simulink model "lab1_simu"  (R2024b)
settings: Solver=VariableStepAuto  StartTime=0.0  StopTime=30  RelTol=1e-3
values from neighbouring files (symbols this model uses):
  A = [0 1 0 0 ... (first row only)    [code_cte_small.m]    (also in lab1.m)
  Afcc = inv(T) * A * T    [code_cte_small.m]    (also in lab1.m)
  Afco = inv(Q)*A*Q    [code_cte_small.m]    (also in lab1.m)
  B = [0 ... (first row only)    [code_cte_small.m]    (also in lab1.m)
  Bfcc = inv(T) * B    [code_cte_small.m]    (also in lab1.m)
  Bfco = inv(Q) * B    [code_cte_small.m]    (also in lab1.m)
  C = [1 0 0 0]    [code_cte_small.m]    (also in lab1.m)
  Cfcc = C * T    [code_cte_small.m]    (also in lab1.m)
  Cfco = C * Q    [code_cte_small.m]    (also in lab1.m)
  E = [0 ... (first row only)    [code_cte_small.m]    (also in lab1.m)
  Efcc = inv(T)*E    [code_cte_small.m]    (also in lab1.m)
  Efco = inv(Q) * E    [code_cte_small.m]    (also in lab1.m)
  KA = [-19.21, 9.68, 4.10, -15.739]    [code_cte_small.m]    (also in lab1.m = [-46190/327, 28467610/962361, -3048419/32700, 2598423281/481)
  KAfcc = [-29798.327,25528.529, 7395.9961,14.998605]    [code_cte_small.m]    (also in lab1.m = [-22691668,516984.21, -10797.714,-24.42])
  kiA = -24.76    [code_cte_small.m]    (also in lab1.m = 67.9102956167)
  kiAfcc = [-151.09413]    [code_cte_small.m]    (also in lab1.m = [67.910289])
settings Model: Creator=Acer  LastModifiedBy=Usuario

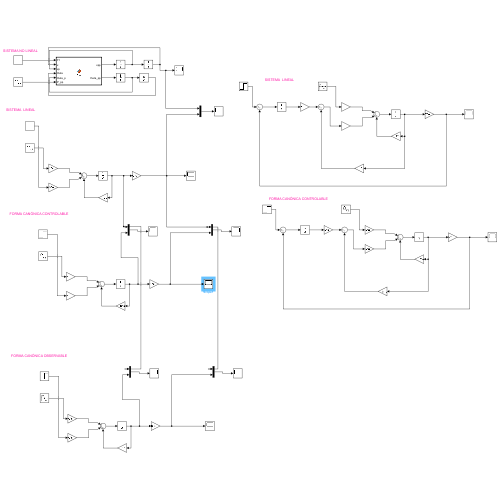
[thumbnail: Simulink's stored preview of the top-level diagram]
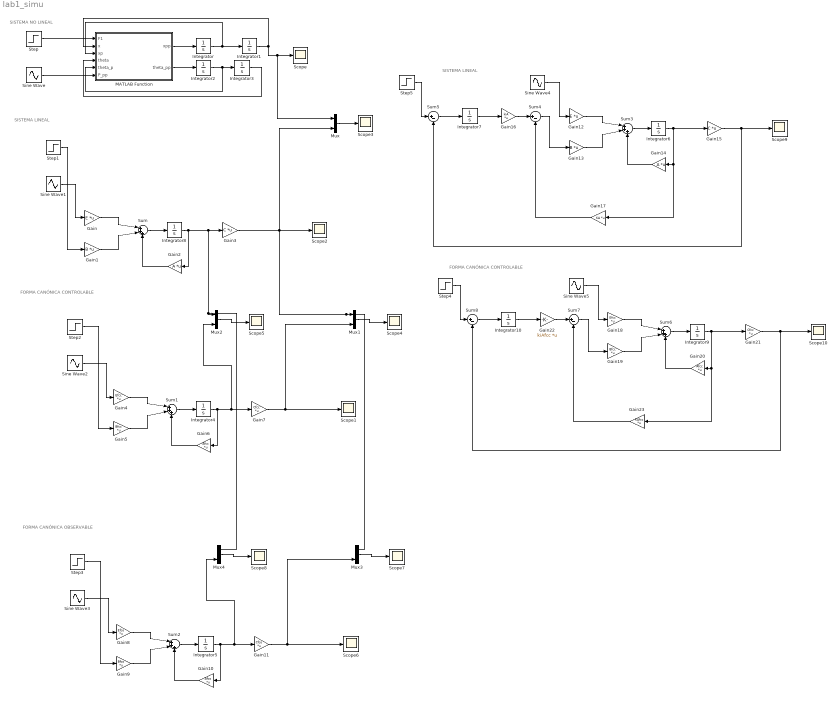
== system lab1_simu ==
  note: SISTEMA LINEAL
  note: SISTEMA NO LINEAL
  note: FORMA CANÓNICA CONTROLABLE
  note: FORMA CANÓNICA OBSERVABLE
  note: SISTEMA LINEAL
  note: FORMA CANÓNICA CONTROLABLE
  Gain : Gain  Gain=E  Multiplication=Matrix(K*u)
  Gain1 : Gain  Gain=B  Multiplication=Matrix(K*u)
  Gain10 : Gain  Gain=Afco  Multiplication=Matrix(K*u)
  Gain11 : Gain  Gain=Cfco  Multiplication=Matrix(K*u)
  Gain12 : Gain  Gain=E  Multiplication=Matrix(K*u)
  Gain13 : Gain  Gain=B  Multiplication=Matrix(K*u)
  Gain14 : Gain  Gain=A  Multiplication=Matrix(K*u)
  Gain15 : Gain  Gain=C  Multiplication=Matrix(K*u)
  Gain16 : Gain  Gain=kiA  Multiplication=Matrix(K*u)
  Gain17 : Gain  Gain=KA  Multiplication=Matrix(K*u)
  Gain18 : Gain  Gain=Efcc  Multiplication=Matrix(K*u)
  Gain19 : Gain  Gain=Bfcc  Multiplication=Matrix(K*u)
  Gain2 : Gain  Gain=A  Multiplication=Matrix(K*u)
  Gain20 : Gain  Gain=Afcc  Multiplication=Matrix(K*u)
  Gain21 : Gain  Gain=Cfcc  Multiplication=Matrix(K*u)
  Gain22 : Gain  Gain=kiAfcc  Multiplication=Matrix(K*u)
  Gain23 : Gain  Gain=KAfcc  Multiplication=Matrix(K*u)
  Gain3 : Gain  Gain=C  Multiplication=Matrix(K*u)
  Gain4 : Gain  Gain=Efcc  Multiplication=Matrix(K*u)
  Gain5 : Gain  Gain=Bfcc  Multiplication=Matrix(K*u)
  Gain6 : Gain  Gain=Afcc  Multiplication=Matrix(K*u)
  Gain7 : Gain  Gain=Cfcc  Multiplication=Matrix(K*u)
  Gain8 : Gain  Gain=Efco  Multiplication=Matrix(K*u)
  Gain9 : Gain  Gain=Bfco  Multiplication=Matrix(K*u)
  Integrator{,1..10} (11 alike) : Integrator
  MATLAB Function : MATLAB Function  TreatAsAtomicUnit=on
  Mux{,1..4} (5 alike) : Mux  Inputs=2
  Scope{,1..10} (11 alike) : Scope
  Sine Wave{,1..5} (6 alike) : Sin  Frequency=5  SampleTime=0
  Step{,1..5} (6 alike) : Step  Time=0  SampleTime=0
  Sum{,1..3,6} (5 alike) : Sum  Inputs=|+++
  Sum{4..5,7..8} (4 alike) : Sum  Inputs=|+-
  wires:
  MATLAB Function/1(xpp) -> Integrator/1
  Integrator/1 -> Integrator1/1, MATLAB Function/3(xp)
  Integrator1/1 -> MATLAB Function/2(x), Mux/1, Scope/1
  MATLAB Function/2(theta_pp) -> Integrator2/1
  Integrator2/1 -> Integrator3/1, MATLAB Function/5(theta_p)
  Integrator3/1 -> MATLAB Function/4(theta)
  Sine Wave/1 -> MATLAB Function/6(P_pp)
  Step/1 -> MATLAB Function/1(F1)
  Step1/1 -> Gain1/1
  Sine Wave1/1 -> Gain/1
  Gain/1 -> Sum/1
  Gain1/1 -> Sum/2
  Sum/1 -> Integrator8/1
  Gain2/1 -> Sum/3
  Integrator8/1 -> Gain2/1, Mux4/1, Mux2/1, Gain3/1
  Gain3/1 -> Mux3/1, Mux1/1, Scope2/1, Mux/2
  Mux/1 -> Scope3/1
  Gain7/1 -> Mux1/2, Scope1/1
  Integrator4/1 -> Mux2/2, Gain7/1, Gain6/1
  Gain6/1 -> Sum1/3
  Sum1/1 -> Integrator4/1
  Gain5/1 -> Sum1/2
  Gain4/1 -> Sum1/1
  Step2/1 -> Gain5/1
  Sine Wave2/1 -> Gain4/1
  Mux1/1 -> Scope4/1
  Mux2/1 -> Scope5/1
  Mux4/1 -> Scope8/1
  Mux3/1 -> Scope7/1
  Sine Wave3/1 -> Gain8/1
  Step3/1 -> Gain9/1
  Gain8/1 -> Sum2/1
  Gain9/1 -> Sum2/2
  Sum2/1 -> Integrator5/1
  Gain10/1 -> Sum2/3
  Integrator5/1 -> Gain10/1, Gain11/1, Mux4/2
  Gain11/1 -> Scope6/1, Mux3/2
  Integrator6/1 -> Gain15/1, Gain17/1, Gain14/1
  Gain14/1 -> Sum3/3
  Sum3/1 -> Integrator6/1
  Gain13/1 -> Sum3/2
  Gain12/1 -> Sum3/1
  Sine Wave4/1 -> Gain12/1
  Step5/1 -> Sum5/1
  Sum5/1 -> Integrator7/1
  Integrator7/1 -> Gain16/1
  Gain16/1 -> Sum4/1
  Gain17/1 -> Sum4/2
  Gain15/1 -> Sum5/2, Scope9/1
  Sum4/1 -> Gain13/1
  Sum7/1 -> Gain19/1
  Gain21/1 -> Scope10/1, Sum8/2
  Gain23/1 -> Sum7/2
  Gain22/1 -> Sum7/1
  Integrator10/1 -> Gain22/1
  Sum8/1 -> Integrator10/1
  Step4/1 -> Sum8/1
  Sine Wave5/1 -> Gain18/1
  Gain18/1 -> Sum6/1
  Gain19/1 -> Sum6/2
  Sum6/1 -> Integrator9/1
  Gain20/1 -> Sum6/3
  Integrator9/1 -> Gain20/1, Gain23/1, Gain21/1

== matlab function lab1_simu/MATLAB Function ==
  data: F1 input; xpp output; x input; xp input; theta input; theta_p input; P_pp input; theta_pp output
function [xpp,theta_pp] = fcn(F1,x,xp, theta,theta_p, P_pp)
k1 = 100;     % N/m
k2 = 150;     % N/m
b1 = 20;   % Ns/m
b2 = 30;   % Ns/m
M  = 2;   % kg
m  = 1;   % kg
g  = 9.81;  % m/s^2
L  = 1;   % m
xpp= (F1-xp*(b1+b2)-x*(k1+k2)+M*g*sin(theta))/m
theta_pp= (-P_pp+((b2+b1)/m)*xp+((k2+k1)/m)*x+((-M/m)-1)*g*sin(theta)-F1)/L;
